simulink model "FINAL_MODEL"  (R2025a)
settings: Solver=FixedStepDiscrete  StartTime=0.0  StopTime=200  FixedStep=0.1  RelTol=1e-3
model workspace (MAT data in the model file):
  P = 1
  W = 1
undefined symbols (not defined in the file): AREA_HELIOS, C, MASS_FULL_TANK, NUMBER_HELIOS, NUMBER_OF_CELLS, POWER_DEMAND, SOLAR_MULTIPLE, SOLAR_PANELS, WIND
settings Model: PacingRate=4  Creator=PARIKSHIT  LastModifiedBy=PARIKSHIT

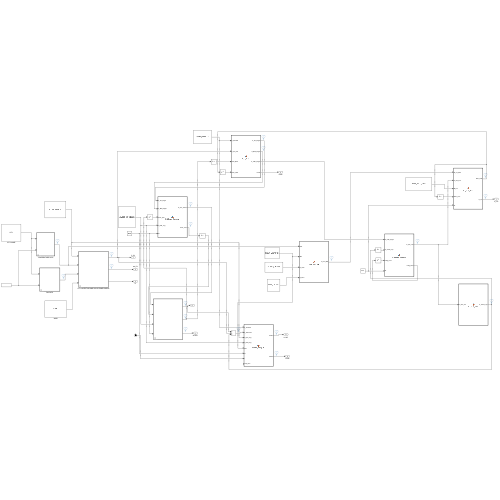
[thumbnail: Simulink's stored preview of the top-level diagram]
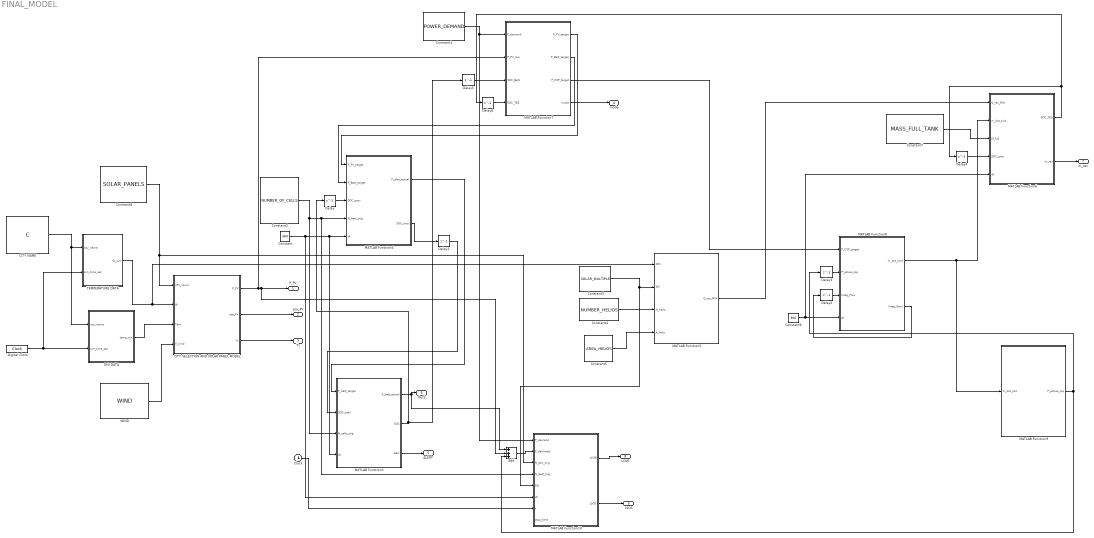
== system FINAL_MODEL ==
  Add : Sum  Inputs=+++
  CITY NAME : Constant  Value=C  VectorParams1D=off
      mask Display: disp('CITY');
  CITY SELECTION AND SOLAR PANEL MODEL : MATLAB Function  TreatAsAtomicUnit=on
  Clock : Clock
  Constant : Constant  Value=360
  Constant1 : Constant  Value=POWER_DEMAND
  Constant2 : Constant  Value=NUMBER_OF_CELLS
  Constant3 : Constant  Value=SOLAR_MULTIPLE
  Constant4 : Constant  Value=NUMBER_HELIOS
  Constant5 : Constant  Value=AREA_HELIOS
  Constant6 : Constant  Value=360
  Constant7 : Constant  Value=MASS_FULL_TANK
  Constant8 : Constant  Value=SOLAR_PANELS
  DNI DATA : MATLAB Function  TreatAsAtomicUnit=on
  Delay{,1..6} (7 alike) : Delay  DelayLength=1  InitialCondition=0
  Digital Clock : DigitalClock
  MATLAB Function10 : MATLAB Function  TreatAsAtomicUnit=on
  MATLAB Function3 : MATLAB Function  TreatAsAtomicUnit=on
  MATLAB Function4 : MATLAB Function  TreatAsAtomicUnit=on
  MATLAB Function5 : MATLAB Function  TreatAsAtomicUnit=on
  MATLAB Function6 : MATLAB Function  TreatAsAtomicUnit=on
  MATLAB Function7 : MATLAB Function  TreatAsAtomicUnit=on
  MATLAB Function8 : MATLAB Function  TreatAsAtomicUnit=on
  MATLAB Function9 : MATLAB Function  TreatAsAtomicUnit=on
  TEMPERATURE DATA : MATLAB Function  TreatAsAtomicUnit=on
  WIND : Constant  Value=WIND
  P_PV : Outport
  eta_PV : Outport  Port=2
  Tc : Outport  Port=3
  mode : Outport  Port=4
  ALERT : Outport  Port=5
  Out2 : Outport  Port=6
  m_rec : Outport  Port=7
  LCOE : Outport  Port=8
  LSOS : Outport  Port=9
  wires:
  DNI DATA/1(temp_out) -> CITY SELECTION AND SOLAR PANEL MODEL/3(Tam)
  Constant8/1 -> MATLAB Function10/3(N_pan_orig), CITY SELECTION AND SOLAR PANEL MODEL/1(nPV_count)
  WIND/1 -> CITY SELECTION AND SOLAR PANEL MODEL/4(V_wind)
  CITY NAME/1 -> DNI DATA/1(city_name), TEMPERATURE DATA/1(city_name)
  Digital Clock/1 -> TEMPERATURE DATA/2(sim_time_sec), DNI DATA/2(sim_time_sec)
  CITY SELECTION AND SOLAR PANEL MODEL/3(Tc) -> Tc/1
  CITY SELECTION AND SOLAR PANEL MODEL/2(eta_PV) -> eta_PV/1
  MATLAB Function3/2(SOC) -> Delay5/1, Delay/1
  Delay/1 -> MATLAB Function4/3(SOC_prev)
  Constant/1 -> MATLAB Function10/6(dt), MATLAB Function3/4(dt), MATLAB Function4/5(dt)
  MATLAB Function7/1(P_PV_target) -> MATLAB Function4/1(P_PV_target)
  MATLAB Function7/2(P_Batt_target) -> MATLAB Function4/2(P_Batt_target)
  Clock/1 -> MATLAB Function10/7(t)
  Constant1/1 -> MATLAB Function10/1(P_demand), MATLAB Function7/1(P_demand)
  CITY SELECTION AND SOLAR PANEL MODEL/1(P_PV) -> MATLAB Function7/2(P_PV_raw), Add/2, P_PV/1
  MATLAB Function6/1(SOC_TES) -> Delay6/1, Delay4/1
  MATLAB Function7/3(P_CSP_target) -> MATLAB Function8/1(P_CSP_target)
  MATLAB Function7/4(mode) -> mode/1
  MATLAB Function3/1(P_batt_actual) -> Out2/1, Add/1
  MATLAB Function4/1(P_elec_actual) -> MATLAB Function3/1(P_batt_target)
  Constant2/1 -> MATLAB Function3/3(N_cells_orig), MATLAB Function10/4(N_batt_orig), MATLAB Function4/4(N_batt_orig)
  MATLAB Function4/2(SOC_next) -> Delay1/1
  Delay1/1 -> MATLAB Function3/2(SOC_prev)
  Constant3/1 -> MATLAB Function10/5(SM), MATLAB Function5/2(SM)
  Constant4/1 -> MATLAB Function5/3(N_helio)
  Constant5/1 -> MATLAB Function5/4(A_helio)
  TEMPERATURE DATA/1(GI_out) -> MATLAB Function5/1(DNI), CITY SELECTION AND SOLAR PANEL MODEL/2(GI)
  MATLAB Function8/2(Integ_Next) -> Delay2/1
  Delay2/1 -> MATLAB Function8/3(Integ_Prev)
  Constant6/1 -> MATLAB Function6/5(dt), MATLAB Function8/4(dt)
  MATLAB Function5/1(Q_rec_MW) -> MATLAB Function6/1(Q_rec_MW)
  MATLAB Function8/1(m_dot_cmd) -> MATLAB Function6/2(m_dot_turb), MATLAB Function9/1(m_dot_co2)
  Constant7/1 -> MATLAB Function6/3(M_full)
  MATLAB Function9/1(P_actual_csp) -> Delay3/1, Add/3
  Delay3/1 -> MATLAB Function8/2(P_actual_csp)
  MATLAB Function6/2(m_rec) -> m_rec/1
  Delay4/1 -> MATLAB Function6/4(SOC_prev)
  MATLAB Function10/1(LCOE) -> LCOE/1
  Add/1 -> MATLAB Function10/2(P_delivered)
  Delay5/1 -> MATLAB Function7/3(SOC_Batt)
  Delay6/1 -> MATLAB Function7/4(SOC_TES)
  MATLAB Function10/2(LSOS) -> LSOS/1
  MATLAB Function3/3(alert) -> ALERT/1

== matlab function FINAL_MODEL/MATLAB Function7 ==
  data: P_demand input; P_PV_raw input; SOC_Batt input; P_PV_target output; P_Batt_target output; SOC_TES input; P_CSP_target output; mode output
function [P_PV_target, P_Batt_target, P_CSP_target, mode] = Major_Brain(P_demand, P_PV_raw, SOC_Batt, SOC_TES)
    % Inputs: MW, MW, 0-1, 0-1
    P_PV_avail = P_PV_raw * 0.98; % Net after inverter
    P_PV_target = 0; P_Batt_target = 0; P_CSP_target = 0; mode = 0;

    if P_PV_avail >= P_demand
        P_PV_target = P_demand;
        mode = 1; % PV covers load
        if SOC_Batt < 0.90
            P_Batt_target = -(P_PV_avail - P_demand); % Charge battery
        end
    else
        P_PV_target = P_PV_avail;
        deficit = P_demand - P_PV_avail;
        if SOC_Batt > 0.15
            P_Batt_target = deficit; % Request from battery
            mode = 2; 
        end
        gap = deficit - max(0, P_Batt_target);
        if gap > 5 && SOC_TES > 0.10
            P_CSP_target = gap;
            mode = 3; % Hybrid Mode
        end
    end
end

== matlab function FINAL_MODEL/MATLAB Function8 ==
  data: P_CSP_target input; m_dot_cmd output; P_actual_csp input; Integ_Prev input; dt input; Integ_Next output
function [m_dot_cmd, Integ_Next] = SubBrain_Thermal(P_CSP_target, P_actual_csp, Integ_Prev, dt)
    eta_cyc = 0.45; Cp = 1.51; dT = 275;
    
    % PID to ensure electrical output matches the dispatcher's target
    error = P_CSP_target - P_actual_csp;
    Integ_Next = Integ_Prev + (error * dt);
    m_correction = (1.2 * error) + (0.3 * Integ_Next);
    
    m_dot_cmd = max(0, min((P_CSP_target/eta_cyc * 1000)/(Cp*dT) + m_correction, 1500));
end

== matlab function FINAL_MODEL/MATLAB Function9 ==
  data: m_dot_co2 input; P_actual_csp output
function P_actual_csp = Physical_sCO2(m_dot_co2)
    % Physics of the Brayton cycle
    eta_turb = 0.90; Cp_co2 = 1.2; Tin = 550; Tout = 410;
    P_kW = m_dot_co2 * Cp_co2 * (Tin - Tout) * eta_turb;
    P_actual_csp = P_kW / 1000; % Convert to MW
end

== matlab function FINAL_MODEL/MATLAB Function10 ==
  data: P_demand input; LCOE output; P_delivered input; N_pan_orig input; N_batt_orig input; SM input; dt input; t input; LSOS output; stop_time input
function [LCOE, LSOS] = Auditor_Analytics(P_demand, P_delivered, N_pan_orig, N_batt_orig, SM, dt, t, stop_time)
    persistent E_gen; 
    persistent E_dem;
    
    if isempty(E_gen) || t <= dt
        E_gen = 1e-6; 
        E_dem = 1e-6;
    end
    
    N_pan_total = N_pan_orig * 10000;
    N_batt_total = N_batt_orig * 10000;
    CAPEX = (N_pan_total * 250) + (N_batt_total * 150) + (SM * 150e6);
    
    E_gen = E_gen + (P_delivered * dt/3600);
    E_dem = E_dem + (P_demand * dt/3600);
    
    LCOE = (CAPEX / 25) / (E_gen / (t/3600 + 0.0001));
    LSOS = max(0, (1 - (E_gen / E_dem)) * 100);
    
    if(E_gen <= 0.01)
        LCOE = -1;
    end
    
    if t >= stop_time - dt
        fprintf('\n========================================\n');
        fprintf('       FINAL SIMULATION RESULTS        \n');
        fprintf('========================================\n');
        fprintf('Total Energy Generated: %.2f MWh\n', E_gen);
        fprintf('Total Energy Demand:    %.2f MWh\n', E_dem);
        fprintf('----------------------------------------\n');
        fprintf('FINAL LCOE:            $%.2f / MWh\n', LCOE);
        fprintf('FINAL LSOS:            %.2f %%\n', LSOS);
        fprintf('========================================\n');
    end
end

== matlab function FINAL_MODEL/DNI DATA ==
  data: city_name input; temp_out output; sim_time_sec input
function temp_out = getCityTemperature(city_name, sim_time_sec)

% Output
temp_out = 0.0;

% Extrinsic
coder.extrinsic('readmatrix','strcat');

% City selection
if city_name == 1
    city = 'Delingha';
elseif city_name == 2
    city = 'Riyadh';
elseif city_name == 3
    city = 'Jhodpur';
elseif city_name == 4
    city = 'Alice';
else
    city = 'Delingha';
end

% Persistent temperature vector
persistent temp_vec

if isempty(temp_vec)
    filename = strcat(city,'_Weather.xlsx');
    data = readmatrix(filename);
    temp_vec = data(1:24, 2);   % 24 samples
end

% One value every 10 seconds
sample_time = 10;   % seconds
idx = floor(sim_time_sec / sample_time) + 1;

% Clamp index WITHOUT length()
if idx < 1
    idx = 1;
elseif idx > 24
    idx = 24;
end
temp_out = temp_vec(idx);

end

== matlab function FINAL_MODEL/CITY SELECTION AND SOLAR PANEL MODEL ==
  data: nPV_count input; P_PV output; GI input; Tam input; V_wind input; eta_PV output; Tc output
function [P_PV, eta_PV, Tc] = SOLAR_PANEL_BLOCK(nPV_count, GI, Tam, V_wind)
    % Parameters... (Keeping your logic exactly as provided)
    nPV_rated = 250; eta_PV_NOM = 0.145; TNOM = 46; Tam_NOM = 20; G_INOM = 800;
    A_MOD = 1.675; gamma = -0.41e-2; f_PV = 0.8; U_NOM = 9.5; tau_alpha = 0.8;
    eta_INV = 0.95; Tc_REF = 25;


    U = 5.7 + 3.8 * V_wind;
    Tc = Tam + ((TNOM - Tam_NOM)/G_INOM) * GI * (U_NOM/U) * (1 - eta_PV_NOM/tau_alpha);
    eta_PV = eta_PV_NOM * (1 + gamma * (Tc - Tc_REF));
    
    % Scaled by 10,000 as requested
    P_DC = nPV_count*10000 * A_MOD * GI * eta_PV * eta_INV * f_PV;
    P_PV = (P_DC * eta_INV)/1000000; % Output in MW

    if GI <= 0, P_PV = 0; eta_PV = 0; end
end

== matlab function FINAL_MODEL/TEMPERATURE DATA ==
  data: city_name input; GI_out output; sim_time_sec input
function GI_out = getCityGI(city_name, sim_time_sec)

% Output
GI_out = 0.0;

% Extrinsic
coder.extrinsic('readmatrix','strcat');
%fprintf("city:%f",city_name);
% City selection
if city_name == 1
    city = 'Delingha';
elseif city_name == 2
    city = 'Riyadh';
elseif city_name == 3
    city = 'Jhodpur';
elseif city_name == 4
    city = 'Alice';
else
    city = 'Delingha';
end

% Persistent GI vector
persistent gi_vec

if isempty(gi_vec)
    filename = strcat(city,'_GI.xlsx');
    data = readmatrix(filename);   % numeric matrix only
    gi_vec = data(1:24, 2);        % 24 GI samples
end

% One value every 10 seconds
sample_time = 10;   % seconds
idx = floor(sim_time_sec / sample_time) + 1;

% Clamp index (NO length())
if idx < 1
    idx = 1;
elseif idx > 24
    idx = 24;
end

% Output scalar GI
GI_out = gi_vec(idx);

end

== matlab function FINAL_MODEL/MATLAB Function3 ==
  data: P_batt_target input; P_batt_actual output; SOC output; alert output; SOC_prev input; N_cells_orig input; dt input
function [P_batt_actual, SOC, alert] = Battery_Model(P_batt_target, SOC_prev, N_cells_orig, dt)
    N_total = N_cells_orig * 10000;
    Eb_max = N_total * 100; % Wh
    Pb_max_W = N_total * 100; % W
    
    Eb = SOC_prev * Eb_max;
    P_req_W = P_batt_target * 1e6; 
    P_batt_actual_W = 0;

    if P_req_W < 0 && SOC_prev < 0.90 % Charge
        P_batt_actual_W = max(P_req_W, -Pb_max_W);
    elseif P_req_W > 0 && SOC_prev > 0.10 % Discharge
        P_batt_actual_W = min(P_req_W, Pb_max_W);
    end

    Eb_next = Eb - (P_batt_actual_W * dt / 3600);
    SOC = max(0.1, min(0.9, Eb_next / Eb_max));
    P_batt_actual = P_batt_actual_W / 1e6;
    alert = (SOC <= 0.1);
end

== matlab function FINAL_MODEL/MATLAB Function4 ==
  data: P_PV_target input; P_elec_actual output; SOC_next output; P_Batt_target input; SOC_prev input; N_batt_orig input; dt input
function [P_elec_actual, SOC_next] = SubBrain_Electrical(P_PV_target, P_Batt_target, SOC_prev, N_batt_orig, dt)
    N_total_batt = N_batt_orig * 10000;
    
    P_batt_max_MW = (N_total_batt * 100) / 1e6;  
    E_batt_cap_MWh = (N_total_batt * 0.4) / 1000; 

    % Charge/Discharge logic
    P_batt_actual = max(min(P_Batt_target, P_batt_max_MW), -P_batt_max_MW);
    
    % Update SOC
    SOC_next = SOC_prev - (P_batt_actual * (dt/3600) / E_batt_cap_MWh);
    SOC_next = max(0.1, min(0.95, SOC_next));
    
    P_elec_actual = P_PV_target + max(0, P_batt_actual);
end

== matlab function FINAL_MODEL/MATLAB Function5 ==
  data: DNI input; Q_rec_MW output; SM input; N_helio input; A_helio input
function Q_rec_MW = Physical_CSP_Field(DNI, SM, N_helio, A_helio)
    eta_field = 0.65; % Optical efficiency
    Q_rec_MW = (DNI * N_helio * A_helio * eta_field * SM) / 1e6;
end

== matlab function FINAL_MODEL/MATLAB Function6 ==
  data: SOC_TES output; Q_rec_MW input; m_rec output; m_dot_turb input; M_full input; SOC_prev input; dt input
function [SOC_TES, m_rec] = Physical_TES(Q_rec_MW, m_dot_turb, M_full, SOC_prev, dt)
    Cp = 1.51; dT = 275;
    m_rec = (Q_rec_MW * 1000) / (Cp * dT); 
    dM = m_rec - m_dot_turb;
    M_new = (SOC_prev * M_full) + (dM * dt);
    SOC_TES = max(0, min(1, M_new / M_full));
end
